simulink model "complete_model"  (R2020b)
settings: Solver=VariableStepAuto  StartTime=0.0  StopTime=10.0  RelTol=1e-3
undefined symbols (not defined in the file or in its folder): D_b_1, D_b_2, D_k_1, D_k_2, D_t_1, D_t_2, E_1, E_2, g, Gs_1, Gs_2, Ix_1, Ix_2, Iy_1, Iy_2, Iz_1, Iz_2, l_1, l_2, m_1, m_2, q_0, q_dot_0
libraries: dspmtrx3 x2, pid_lib x1, dspinverses x1
(part 1 of 2)
settings Model: Creator=lucar  LastModifiedBy=lucar

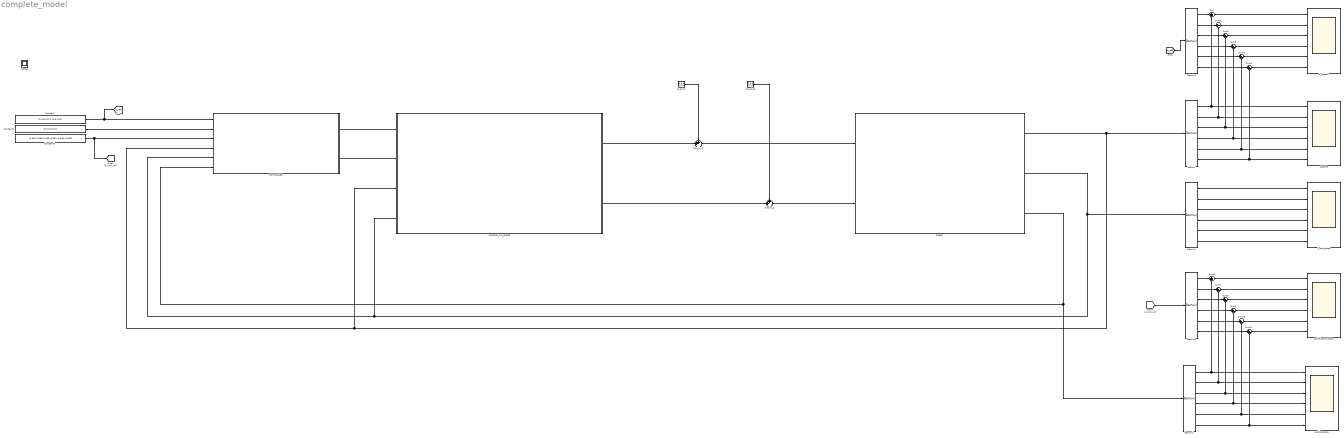
== system complete_model ==
  CONTROLLER : Subsystem
  "CONTROL_TO_FORCE " : Subsystem
  Constant : Constant  Value=[1 0.5 0.3 -1 -0.5 -0.3]
  Constant3 : Constant  Value=[0.001 0.008 0.003 -0.001 -0.005 -0.003]
  Constant4 : Constant  Value=[0 0 0 0 0 0]
  Demux{,1..3,5} (5 alike) : Demux  Outputs=6
  ROBOT : Subsystem
  SUM_W_1 : Sum  Inputs=++|
  SUM_W_2 : Sum  Inputs=++|
  Sum{,1..11} (12 alike) : Sum  Inputs=|+-
  W_ext_1 : Constant  Value=[0 0 0 0 0 0]
  W_ext_21 : Constant  Value=[0 0 0 0 0 0]
  q_ddot_error_scope : Scope  NumInputPorts=6
  q_ddot_scope : Scope  NumInputPorts=6
  q_dot_scope : Scope  NumInputPorts=6
  q_scope : Scope  NumInputPorts=6
  q_scope1 : Scope  NumInputPorts=6
  Scope : Scope
  wires:
  Constant4/1 -> CONTROLLER/2(q_dot_ref)
  "CONTROL_TO_FORCE "/1(W_ctrl_1) -> SUM_W_1/2
  ROBOT/1(q) -> Demux/1, "CONTROL_TO_FORCE "/3(q), CONTROLLER/4(q)
  W_ext_1/1 -> SUM_W_1/1
  W_ext_21/1 -> SUM_W_2/1
  CONTROLLER/1(u_control_1) -> "CONTROL_TO_FORCE "/1(u_ctrl_1)
  CONTROLLER/2(u_control_2) -> "CONTROL_TO_FORCE "/2(u_ctrl_2)
  Constant/1 -> [q_ref], CONTROLLER/1(q_ref)
  SUM_W_2/1 -> ROBOT/2(W2)
  SUM_W_1/1 -> ROBOT/1(W_1)
  "CONTROL_TO_FORCE "/2(W_ctrl_2) -> SUM_W_2/2
  Demux/2 -> q_scope/2, Sum1/2  "b_1"
  Demux/1 -> Sum/2, q_scope/1  "k_1"
  Demux/3 -> q_scope/3, Sum2/2  "t_1"
  Demux/4 -> q_scope/4, Sum3/2  "k_2"
  Demux/5 -> q_scope/5, Sum4/2  "b_2"
  Demux/6 -> q_scope/6, Sum5/2  "t_2"
  Demux1/1 -> q_dot_scope/1  "k_1_dot"
  Demux1/5 -> q_dot_scope/5  "b_2_dot"
  ROBOT/2(q_dot) -> Demux1/1, "CONTROL_TO_FORCE "/4(q_dot), CONTROLLER/5(q_dot)
  Demux1/4 -> q_dot_scope/4  "k_2_dot"
  Demux1/3 -> q_dot_scope/3  "t_1_dot"
  Demux1/2 -> q_dot_scope/2  "b_1_dot"
  Demux1/6 -> q_dot_scope/6  "t_2_dopt"
  Demux3/2 -> Sum1/1  "b_1"
  Demux3/1 -> Sum/1  "k_1"
  Demux3/3 -> Sum2/1  "t_1"
  Demux3/6 -> Sum5/1  "t_2"
  Demux3/4 -> Sum3/1  "k_2"
  Demux3/5 -> Sum4/1  "b_2"
  [q_ref] -> Demux3/1
  Sum5/1 -> q_scope1/6
  Sum4/1 -> q_scope1/5
  Sum3/1 -> q_scope1/4
  Sum2/1 -> q_scope1/3
  Sum1/1 -> q_scope1/2  "b_1_error"
  Sum/1 -> q_scope1/1  "k_1_error"
  ROBOT/3(q_ddot) -> Demux2/1, CONTROLLER/6(q_ddot)
  Demux5/4 -> Sum9/1  "k_2"
  Sum6/1 -> q_ddot_error_scope/1  "k_1_ddot_error"
  Demux5/2 -> Sum7/1  "b_1"
  Demux5/6 -> Sum11/1  "t_2"
  Sum11/1 -> q_ddot_error_scope/6  "t_2_ddot_error"
  Sum9/1 -> q_ddot_error_scope/4  "k_2_ddot_error"
  Demux5/5 -> Sum10/1  "b_2"
  Demux5/3 -> Sum8/1  "t_1"
  Sum8/1 -> q_ddot_error_scope/3  "t_1_ddot_error"
  Sum10/1 -> q_ddot_error_scope/5  "b_2_ddot_error"
  Demux5/1 -> Sum6/1  "k_1"
  Sum7/1 -> q_ddot_error_scope/2  "b_1_ddot_error"
  Demux2/5 -> q_ddot_scope/5, Sum10/2  "b_2_ddot"
  Demux2/3 -> q_ddot_scope/3, Sum8/2  "t_1_ddot"
  Demux2/1 -> q_ddot_scope/1, Sum6/2  "k_1_ddot"
  Demux2/6 -> q_ddot_scope/6, Sum11/2  "t_2_ddot"
  Demux2/2 -> q_ddot_scope/2, Sum7/2  "b_1_ddot"
  Demux2/4 -> q_ddot_scope/4, Sum9/2  "k_2_ddot"
  Constant3/1 -> [q_ddot_ref], CONTROLLER/3(q_ddot_ref)
  [q_ddot_ref] -> Demux5/1

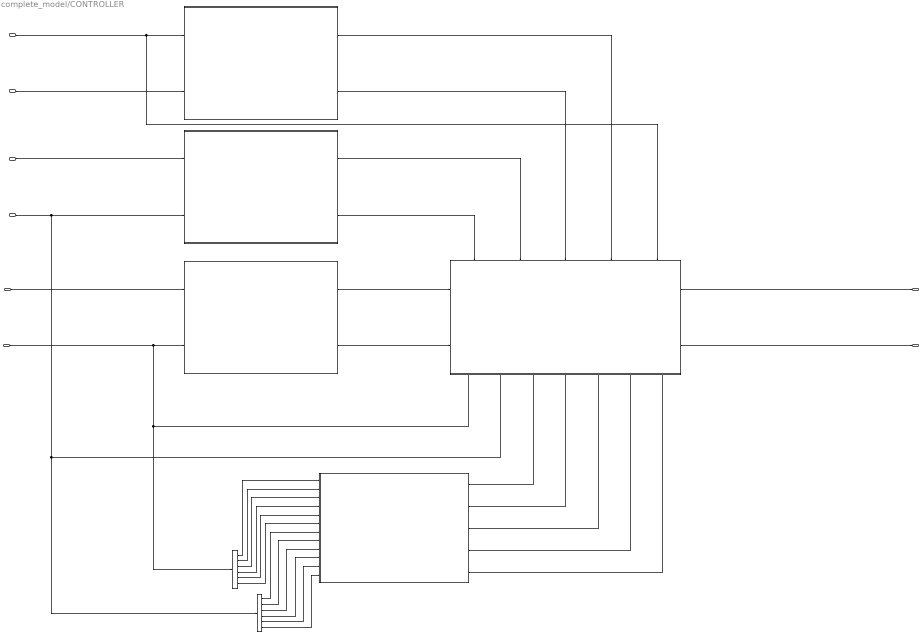
== system complete_model/CONTROLLER ==
  q_ref : Inport
  q_dot_ref : Inport  Port=2
  q_ddot_ref : Inport  Port=3
  q : Inport  Port=4
  q_dot : Inport  Port=5
  q_ddot : Inport  Port=6
  Demux2 : Demux  Outputs=6
  Demux3 : Demux  Outputs=6
  Subsystem : Subsystem
  Subsystem1 : Subsystem
      settings: PortSchema="{\"entries\":[{\"content\":{\"sides\":[{\"content\":{\"connectorIds\":[\"In1\",\"In2\"]},\"type\":\"ConnectorPlacement.EquallySpacedRectSide\",\"uuid\":\"f5a8289a-49c1-4c4e-8602-865d2a4ae65f\"},{\"content\":{\"connectorIds\":[\"Out1\",\"Out2\"],\"side\":\"RIGHT\"},\"type\":\"ConnectorPlacement.EquallySpacedRectSide\",\"uuid\":\"577a7826-c2f6-45a0-b52d-c6289559e493\"},{\"content\":{\"connectorIds\":[\"In3\",\"In4\",\"In5\",\"In6\",\"In7\"],\"side\":\"TOP\"},\"type\":\"ConnectorPlacement.EquallySpacedRectSide\",\"uuid\":\"a36ac755-a99f-4894-9541-2e1b1dc6ecfa\"},{\"content\":{\"connectorIds\":[\"In8\",\"In9\",\"In10\",\"In11\",\"In12\",\"In13\",\"In14\"],\"side\":\"BOTTOM\"},\"type\":\"ConnectorPlacement.EquallySpacedRectSide\",\"uuid\":\"cdbb495b-8222-4370-93c0-90b4d729da35\"},{\"content\":{\"connectorIds\":[],\"side\":\"HIDDEN\"},\"type\":\"ConnectorPlacement.EquallySpacedRectSide\",\"uuid\":\"56f17497-4814-45df-afce-b6f00d804874\"}]},\"type\":\"ConnectorPlacement.EquallySpacedConnector\",\"uuid\":\"c7bc0292-f10c-440d-b55e-954c700d4dfb\"}],\"packageUris\":[\"http://schema.mathworks.com/mf0/Connector/R2020b\"],\"version\":\"1.0\"}"
  Subsystem2 : Subsystem
  Subsystem3 : Subsystem
  Subsystem4 : Subsystem
  u_control_1 : Outport
  u_control_2 : Outport  Port=2
  wires:
  q_ref/1 -> Subsystem/1(In1)
  Subsystem/1(e_1) -> Subsystem1/1(e_1)
  Subsystem/2(e_2) -> Subsystem1/2(e_2)
  Subsystem1/1(u_control_1) -> u_control_1/1
  Subsystem1/2(u_control_2) -> u_control_2/1
  Demux2/6 -> Subsystem2/6(t_2)
  q/1 -> Subsystem/2(In2), Subsystem1/8(q), Demux2/1
  Demux3/3 -> Subsystem2/9(t_dot_1)
  Demux3/1 -> Subsystem2/7(k_dot_1)
  Demux3/2 -> Subsystem2/8(b_dot_1)
  Demux2/4 -> Subsystem2/4(k_2)
  Demux2/2 -> Subsystem2/2(b_1)
  Demux2/1 -> Subsystem2/1(k_1)
  Demux2/3 -> Subsystem2/3(t_1)
  Demux3/5 -> Subsystem2/11(b_dot_2)
  q_dot/1 -> Subsystem1/9(q_dot), Demux3/1, Subsystem3/2(q_dot)
  Demux2/5 -> Subsystem2/5(b_2)
  Demux3/4 -> Subsystem2/10(k_dot_2)
  Demux3/6 -> Subsystem2/12(t_dot_2)
  Subsystem2/1(B) -> Subsystem1/10(B)
  Subsystem2/2(D) -> Subsystem1/11(D)
  Subsystem2/3(C) -> Subsystem1/12(C)
  Subsystem2/4(G) -> Subsystem1/13(G)
  q_dot_ref/1 -> Subsystem3/1(q_dot_ref)
  q_ddot_ref/1 -> Subsystem1/7(q_ddot_ref), Subsystem4/1(q_ddot_ref)
  q_ddot/1 -> Subsystem4/2(q_ddot)
  Subsystem3/2(e_2) -> Subsystem1/3(e_dot_1)
  Subsystem3/1(e_1) -> Subsystem1/4(e_dot_2)
  Subsystem4/2(e_ddot_2) -> Subsystem1/5(e_ddot_1)
  Subsystem4/1(e_ddot_1) -> Subsystem1/6(e_ddot_2)
  Subsystem2/5(G_grav) -> Subsystem1/14(G_grav)

== system complete_model/CONTROL_TO_FORCE  ==
  u_ctrl_1 : Inport
  u_ctrl_2 : Inport  Port=2
  q : Inport  Port=3
  q_dot : Inport  Port=4
  Demux : Demux  Outputs=6
  Demux1 : Demux  Outputs=6
  Subsystem : Subsystem
  W_ctrl_1 : Outport
  W_ctrl_2 : Outport  Port=2
  wires:
  Demux/6 -> Subsystem/8(t_2)
  q/1 -> Demux/1
  Demux1/3 -> Subsystem/11(t_dot_1)
  Demux1/1 -> Subsystem/9(k_dot_1)
  Demux1/2 -> Subsystem/10(b_dot_1)
  Demux/4 -> Subsystem/6(k_2)
  Demux/2 -> Subsystem/4(b_1)
  Demux/1 -> Subsystem/3(k_1)
  Demux/3 -> Subsystem/5(t_1)
  Demux1/5 -> Subsystem/13(b_dot_2)
  q_dot/1 -> Demux1/1
  Demux/5 -> Subsystem/7(b_2)
  Demux1/4 -> Subsystem/12(k_dot_2)
  Demux1/6 -> Subsystem/14(t_dot_2)
  Subsystem/1(W_ctrl_1) -> W_ctrl_1/1
  Subsystem/2(W_ctrl_2) -> W_ctrl_2/1
  u_ctrl_1/1 -> Subsystem/1(u_ctrl_1)
  u_ctrl_2/1 -> Subsystem/2(u_ctrl_2)

== system complete_model/ROBOT ==
  W_1 : Inport
  W2 : Inport  Port=2
  Demux : Demux  Outputs=6
  Demux1 : Demux  Outputs=6
  Integrator : Integrator  InitialCondition=q_dot_0
  Integrator1 : Integrator  InitialCondition=q_0
  Subsystem : Subsystem
  Subsystem1 : Subsystem
  q : Outport
  q_dot : Outport  Port=2
  q_ddot : Outport  Port=3
  wires:
  Subsystem/4(G) -> Subsystem1/5(G)
  Demux/3 -> Subsystem/3(t_1)
  Demux1/6 -> Subsystem/14(t_dot_2)
  Demux1/5 -> Subsystem/13(b_dot_2)
  Demux1/2 -> Subsystem/10(b_dot_1)
  Demux1/4 -> Subsystem/12(k_dot_2)
  Demux/5 -> Subsystem/5(b_2)
  Demux/1 -> Subsystem/1(k_1)
  Subsystem1/1(q_ddot) -> q_ddot/1, Integrator/1
  Demux/4 -> Subsystem/4(k_2)
  Demux1/3 -> Subsystem/11(t_dot_1)
  Demux/2 -> Subsystem/2(b_1)
  Subsystem/1(B) -> Subsystem1/2(B)
  Demux1/1 -> Subsystem/9(k_dot_1)
  Subsystem/3(C) -> Subsystem1/4(C)
  Demux/6 -> Subsystem/6(t_2)
  Subsystem/2(D) -> Subsystem1/3(D)
  W_1/1 -> Subsystem/7(W_1)
  Subsystem/5(U) -> Subsystem1/6(u)
  W2/1 -> Subsystem/8(W_2)
  Integrator1/1 -> q/1, Subsystem1/1(q), Demux/1
  Integrator/1 -> Demux1/1, Subsystem1/7(q_dot), Integrator1/1, q_dot/1

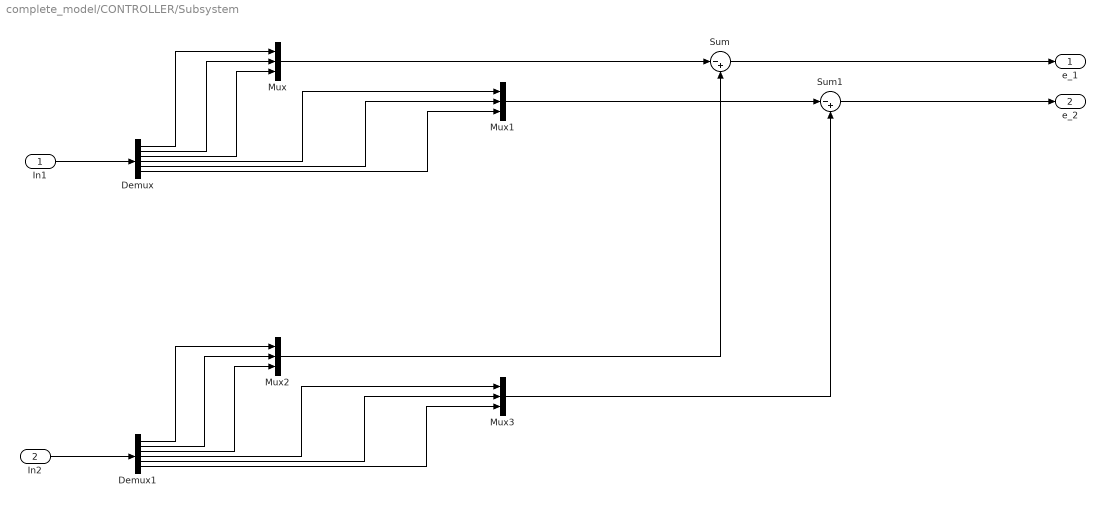
== system complete_model/CONTROLLER/Subsystem ==
  In1 : Inport
  In2 : Inport  Port=2
  Demux : Demux  Outputs=6
  Demux1 : Demux  Outputs=6
  Mux{,1..3} (4 alike) : Mux  Inputs=3
  Sum : Sum  Inputs=|-+
  Sum1 : Sum  Inputs=|-+
  e_1 : Outport
  e_2 : Outport  Port=2
  wires:
  Demux1/6 -> Mux3/3
  Demux/3 -> Mux/3
  Demux1/5 -> Mux3/2
  Demux/2 -> Mux/2
  Mux2/1 -> Sum/2
  Demux/6 -> Mux1/3
  Sum1/1 -> e_2/1
  Demux/1 -> Mux/1
  Demux1/4 -> Mux3/1
  Demux1/3 -> Mux2/3
  Demux1/2 -> Mux2/2
  Demux/5 -> Mux1/2
  Demux1/1 -> Mux2/1
  Sum/1 -> e_1/1
  Mux1/1 -> Sum1/1
  Demux/4 -> Mux1/1
  Mux3/1 -> Sum1/2
  Mux/1 -> Sum/1
  In1/1 -> Demux/1
  In2/1 -> Demux1/1

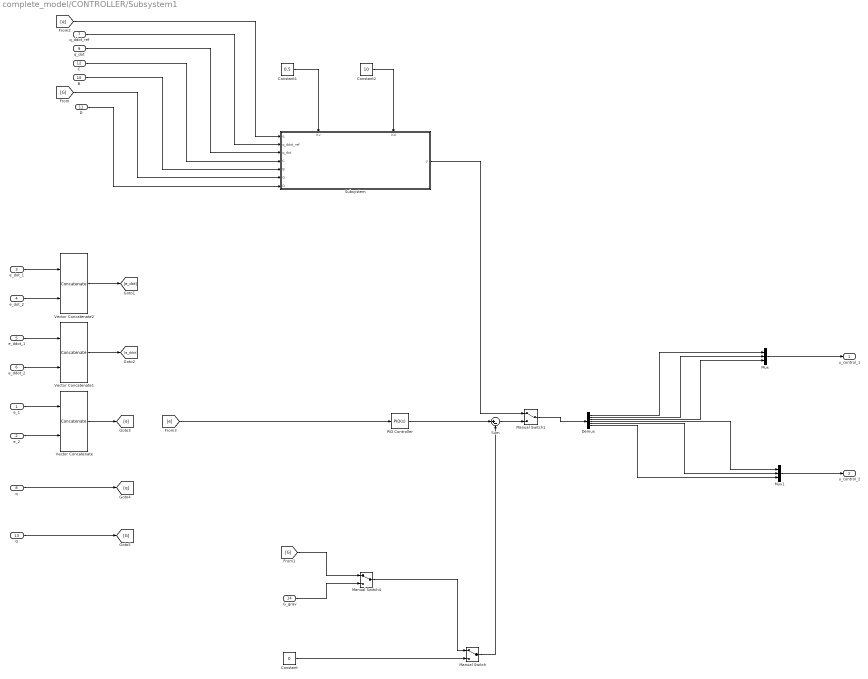
== system complete_model/CONTROLLER/Subsystem1 ==
  e_1 : Inport
  e_2 : Inport  Port=2
  e_dot_1 : Inport  Port=3
  e_dot_2 : Inport  Port=4
  e_ddot_1 : Inport  Port=5
  e_ddot_2 : Inport  Port=6
  q_ddot_ref : Inport  Port=7
  q : Inport  Port=8
  q_dot : Inport  Port=9
  B : Inport  Port=10
  D : Inport  Port=11
  C : Inport  Port=12
  G : Inport  Port=13
  G_grav : Inport  Port=14
  Constant : Constant  Value=0
  Constant1 : Constant  Value=0.5
  Constant2 : Constant  Value=10
  Demux : Demux  Outputs=6
  Manual Switch : ManualSwitch
  Manual Switch1 : ManualSwitch
  Manual Switch4 : ManualSwitch
  Mux : Mux  Inputs=3
  Mux1 : Mux  Inputs=3
  PID Controller : pid_lib/PID Controller  Controller=PID  Form=Parallel  TimeDomain=Continuous-time  UseExternalTs=off  SampleTime=-1  IntegratorMethod=Forward Euler  FilterMethod=Forward Euler  ControllerParametersSource=internal  P=10  I=0  D=0.8  UseFilter=on  N=100  TunerSelectOption=Transfer Function Based (PID Tuner App)  InitialConditionSource=internal  InitialConditionForIntegrator=0  InitialConditionForFilter=0  DifferentiatorICPrevScaledInput=0  ExternalReset=none  TrackingMode=off  Kt=1  LimitOutput=off  SatLimitsSource=internal  UpperSaturationLimit=inf  LowerSaturationLimit=-inf  LinearizeAsGain=on  AntiWindupMode=none  Kb=1  POutMin=[]  POutMax=[]  IOutMin=[]  IOutMax=[]  DOutMin=[]  DOutMax=[]  NOutMin=[]  NOutMax=[]  SumOutMin=[]  SumOutMax=[]  SaturationOutMin=[]  SaturationOutMax=[]  PParamMin=[]  PParamMax=[]  IParamMin=[]  IParamMax=[]  DParamMin=[]  DParamMax=[]  NParamMin=[]  NParamMax=[]  KbParamMin=[]  KbParamMax=[]  KtParamMin=[]  KtParamMax=[]  KbOutMin=[]  KbOutMax=[]  KtOutMin=[]  KtOutMax=[]  IntegratorOutMin=[]  IntegratorOutMax=[]  FilterOutMin=[]  FilterOutMax=[]  SumI1OutMin=[]  SumI1OutMax=[]  SumI2OutMin=[]  SumI2OutMax=[]  SumI3OutMin=[]  SumI3OutMax=[]  SumI4OutMin=[]  SumI4OutMax=[]  SumDOutMin=[]  SumDOutMax=[]  DifferentiatorOutMin=[]  DifferentiatorOutMax=[]  FilterDiffOutCoefMin=[]  FilterDiffOutCoefMax=[]  ReciprocalOutMin=[]  ReciprocalOutMax=[]  SumDenOutMin=[]  SumDenOutMax=[]  SumNumOutMin=[]  SumNumOutMax=[]  DivideOutMin=[]  DivideOutMax=[]  UdiffTsProdOutMin=[]  UdiffTsProdOutMax=[]  NTsProdOutMin=[]  NTsProdOutMax=[]  UintegralTsProdOutMin=[]  UintegralTsProdOutMax=[]  UngainTsProdOutMin=[]  UngainTsProdOutMax=[]  IntegratorContinuousStateAttributes=''  IntegratorStateMustResolveToSignalObject=off  IntegratorRTWStateStorageClass=Auto  FilterContinuousStateAttributes=''  FilterStateMustResolveToSignalObject=off  FilterRTWStateStorageClass=Auto  ParallelPVariant=InternalParameters  IdealPVariant=Disabled  IVariant=InternalParameters  DVariant=InternalParameters  IntegratorVariant=Continuous  SatVariant=Disabled  AWVariant=Passthrough  PCopyVariant=Disabled  TRVariant=Disabled  FdbkBlocksVariant=Forward  IdealPFdbkVariant=Disabled  SatFdbkVariant=Disabled  DerivativeFilterVariant=ContFilter  NVariant=InternalParameters  NCopyVariant=Disabled  FilterICVariant=InternalICsFilter  IntegratorICVariant=InternalICs  ExternalResetVariant=Disabled  TRSumVariant=Passthrough  SumFdbkVariant=Disabled  SumVariant=Sum_PID  TsampFilterVariant=InternalTs  TsampNgainVariant=Passthrough  TsampIntegralVariant=Passthrough  ExternalSaturationOutDataTypeStr=Inherit: Same as second input
  Subsystem : Subsystem
      settings: PortSchema="{\"entries\":[{\"content\":{\"sides\":[{\"content\":{\"connectorIds\":[\"In1\",\"In2\",\"In3\",\"In4\",\"In5\",\"In6\",\"In7\"]},\"type\":\"ConnectorPlacement.EquallySpacedRectSide\",\"uuid\":\"f8378435-2c70-4ca5-b35e-9079000a7188\"},{\"content\":{\"connectorIds\":[\"Out1\"],\"side\":\"RIGHT\"},\"type\":\"ConnectorPlacement.EquallySpacedRectSide\",\"uuid\":\"366e5ae4-a472-4777-8df5-111cdf47ee59\"},{\"content\":{\"connectorIds\":[\"In8\",\"In9\"],\"side\":\"TOP\"},\"type\":\"ConnectorPlacement.EquallySpacedRectSide\",\"uuid\":\"5a70f401-e563-4b1e-a39f-751f70217f1b\"},{\"content\":{\"connectorIds\":[],\"side\":\"HIDDEN\"},\"type\":\"ConnectorPlacement.EquallySpacedRectSide\",\"uuid\":\"6db507d4-eb44-4222-b62b-10b8d3c8cf59\"}]},\"type\":\"ConnectorPlacement.EquallySpacedConnector\",\"uuid\":\"f0240563-1769-4d53-af5c-dad4dbe59b0a\"}],\"packageUris\":[\"http://schema.mathworks.com/mf0/Connector/R2020b\"],\"version\":\"1.0\"}"
  Sum : Sum  Inputs=|+-
  Vector Concatenate : Concatenate
  Vector Concatenate1 : Concatenate
  Vector Concatenate2 : Concatenate
  u_control_1 : Outport
  u_control_2 : Outport  Port=2
  wires:
  e_1/1 -> Vector Concatenate/1
  e_2/1 -> Vector Concatenate/2
  Demux/3 -> Mux/3
  Demux/2 -> Mux/2
  Mux/1 -> u_control_1/1
  Demux/5 -> Mux1/2
  Mux1/1 -> u_control_2/1
  Demux/6 -> Mux1/3
  Demux/1 -> Mux/1
  Demux/4 -> Mux1/1
  Sum/1 -> Manual Switch1/2
  Manual Switch/1 -> Sum/2
  Manual Switch4/1 -> Manual Switch/1
  Constant/1 -> Manual Switch/2
  e_ddot_2/1 -> Vector Concatenate1/2
  e_ddot_1/1 -> Vector Concatenate1/1
  e_dot_2/1 -> Vector Concatenate2/2
  e_dot_1/1 -> Vector Concatenate2/1
  PID Controller/1 -> Sum/1
  Vector Concatenate2/1 -> [e_dot]
  Vector Concatenate1/1 -> [e_ddot]
  Manual Switch1/1 -> Demux/1
  Vector Concatenate/1 -> [e]
  [e] -> PID Controller/1
  q_ddot_ref/1 -> Subsystem/2(q_ddot_ref)
  q_dot/1 -> Subsystem/3(q_dot)
  C/1 -> Subsystem/4(C)
  B/1 -> Subsystem/5(B)
  [G] -> Subsystem/6(G)
  D/1 -> Subsystem/7(D)
  Subsystem/1(y) -> Manual Switch1/1
  Constant1/1 -> Subsystem/8(Kv)
  Constant2/1 -> Subsystem/9(Kd)
  [G] -> Manual Switch4/1
  G_grav/1 -> Manual Switch4/2
  G/1 -> [G]
  q/1 -> [q]
  [q] -> Subsystem/1(q)

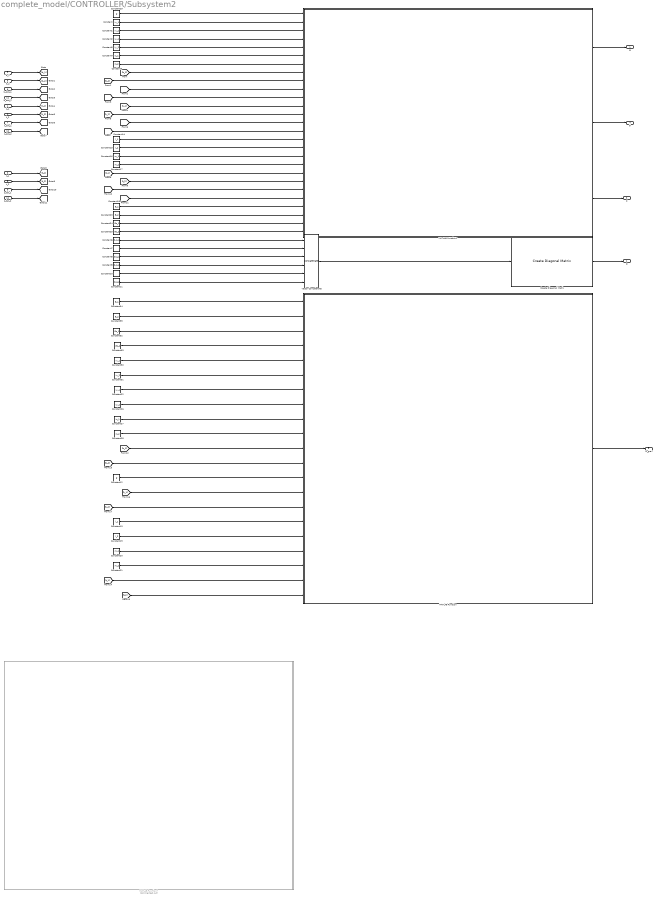
== system complete_model/CONTROLLER/Subsystem2 ==
  k_1 : Inport
  b_1 : Inport  Port=2
  t_1 : Inport  Port=3
  k_2 : Inport  Port=4
  b_2 : Inport  Port=5
  t_2 : Inport  Port=6
  k_dot_1 : Inport  Port=7
  b_dot_1 : Inport  Port=8
  t_dot_1 : Inport  Port=9
  k_dot_2 : Inport  Port=10
  b_dot_2 : Inport  Port=11
  t_dot_2 : Inport  Port=12
  Constant : Constant  Value=Ix_1
  Constant1 : Constant  Value=Ix_2
  Constant10 : Constant  Value=D_b_2
  Constant11 : Constant  Value=D_t_2
  Constant12 : Constant  Value=g
  Constant13 : Constant  Value=l_1
  Constant14 : Constant  Value=l_1
  Constant15 : Constant  Value=l_2
  Constant16 : Constant  Value=m_1
  Constant17 : Constant  Value=m_2
  Constant18 : Constant  Value=E_1
  Constant19 : Constant  Value=l_2
  Constant2 : Constant  Value=Iy_1
  Constant20 : Constant  Value=m_1
  Constant21 : Constant  Value=m_2
  Constant22 : Constant  Value=Iy_1
  Constant23 : Constant  Value=E_2
  Constant24 : Constant  Value=Gs_1
  Constant25 : Constant  Value=Gs_2
  Constant26 : Constant  Value=Iy_2
  Constant27 : Constant  Value=Iz_1
  Constant28 : Constant  Value=Iz_2
  Constant29 : Constant  Value=g
  Constant3 : Constant  Value=Iy_2
  Constant30 : Constant  Value=Ix_1
  Constant31 : Constant  Value=Ix_2
  Constant32 : Constant  Value=Gs_1
  Constant33 : Constant  Value=Gs_2
  Constant34 : Constant  Value=E_1
  Constant35 : Constant  Value=E_2
  Constant4 : Constant  Value=Iz_1
  Constant5 : Constant  Value=Iz_2
  Constant6 : Constant  Value=D_k_1
  Constant7 : Constant  Value=D_b_1
  Constant8 : Constant  Value=D_t_1
  Constant9 : Constant  Value=D_k_2
  Create Diagonal Matrix : dspmtrx3/Create Diagonal Matrix
      settings: SourceProductBaseCode=DS
  MATLAB Function : MATLAB Function  TreatAsAtomicUnit=on
  MATLAB Function1 : Subsystem
      mask help: Simulink:masks:GenSFuncDesc_MD
      mask Help: eval('feval(''rtwprivate'',''rtwhelpview'',''rtw_sfcn_block'')');
  MATLAB Function2 : MATLAB Function  Commented=on  TreatAsAtomicUnit=on
  Vector Concatenate : Concatenate  NumInputs=6
  B : Outport
  D : Outport  Port=2
  C : Outport  Port=3
  G : Outport  Port=4
  G_grav : Outport  Port=5
  wires:
  MATLAB Function1/3(C_matrix) -> C/1
  Constant5/1 -> MATLAB Function1/7(Iz_2)
  Constant18/1 -> MATLAB Function1/24(E_1)
  Constant16/1 -> MATLAB Function1/18(m_1)
  Constant17/1 -> MATLAB Function1/19(m_2)
  Constant25/1 -> MATLAB Function1/27(Gs_2)
  Constant14/1 -> MATLAB Function1/16(l_1)
  Constant1/1 -> MATLAB Function1/3(Ix_2)
  Constant/1 -> MATLAB Function1/2(Ix_1)
  Constant3/1 -> MATLAB Function1/5(Iy_2)
  Constant2/1 -> MATLAB Function1/4(Iy_1)
  Constant4/1 -> MATLAB Function1/6(Iz_1)
  Constant29/1 -> MATLAB Function1/1(g)
  Constant24/1 -> MATLAB Function1/26(Gs_1)
  Constant23/1 -> MATLAB Function1/25(E_2)
  Constant15/1 -> MATLAB Function1/17(l_2)
  MATLAB Function1/1(B_matrix) -> B/1
  MATLAB Function1/2(G_matrix) -> G/1
  Constant7/1 -> Vector Concatenate/2
  Constant6/1 -> Vector Concatenate/1
  Constant8/1 -> Vector Concatenate/3
  Constant9/1 -> Vector Concatenate/4
  Constant10/1 -> Vector Concatenate/5
  Constant11/1 -> Vector Concatenate/6
  Vector Concatenate/1 -> Create Diagonal Matrix/1
  Create Diagonal Matrix/1 -> D/1
  b_1/1 -> [b_1]
  b_2/1 -> [b_2]
  b_dot_1/1 -> [b_dot_1]
  b_dot_2/1 -> [b_dot_2]
  k_1/1 -> [k_1]
  k_2/1 -> [k_2]
  k_dot_1/1 -> [k_dot_1]
  k_dot_2/1 -> [k_dot_2]
  t_2/1 -> [t_2]
  t_dot_2/1 -> [t_dot_2]
  t_1/1 -> [t_1]
  t_dot_1/1 -> [t_dot_1]
  [b_1] -> MATLAB Function1/8(b_1)
  [b_dot_2] -> MATLAB Function1/11(b_dot_2)
  [b_2] -> MATLAB Function1/9(b_2)
  [b_dot_1] -> MATLAB Function1/10(b_dot_1)
  [k_1] -> MATLAB Function1/12(k_1)
  [k_dot_1] -> MATLAB Function1/14(k_dot_1)
  [k_2] -> MATLAB Function1/13(k_2)
  [k_dot_2] -> MATLAB Function1/15(k_dot_2)
  [t_dot_2] -> MATLAB Function1/23(t_dot_2)
  [t_2] -> MATLAB Function1/21(t_2)
  [t_dot_1] -> MATLAB Function1/22(t_dot_1)
  [t_1] -> MATLAB Function1/20(t_1)
  [b_2] -> MATLAB Function/12(b_2)
  [b_1] -> MATLAB Function/11(b_1)
  [t_2] -> MATLAB Function/21(t_2)
  [t_1] -> MATLAB Function/20(t_1)
  Constant12/1 -> MATLAB Function/13(g)
  [k_1] -> MATLAB Function/14(k_1)
  [k_2] -> MATLAB Function/15(k_2)
  Constant19/1 -> MATLAB Function/17(l_2)
  Constant13/1 -> MATLAB Function/16(l_1)
  Constant20/1 -> MATLAB Function/18(m_1)
  Constant21/1 -> MATLAB Function/19(m_2)
  Constant28/1 -> MATLAB Function/10(Iz_2)
  Constant27/1 -> MATLAB Function/9(Iz_1)
  Constant26/1 -> MATLAB Function/8(Iy_2)
  Constant22/1 -> MATLAB Function/7(Iy_1)
  Constant31/1 -> MATLAB Function/6(Ix_2)
  Constant30/1 -> MATLAB Function/5(Ix_1)
  Constant32/1 -> MATLAB Function/3(Gs_1)
  Constant33/1 -> MATLAB Function/4(Gs_2)
  Constant34/1 -> MATLAB Function/1(E_1)
  Constant35/1 -> MATLAB Function/2(E_2)
  MATLAB Function/1(G_g) -> G_grav/1

== system complete_model/CONTROLLER/Subsystem3 ==
  q_dot_ref : Inport
  q_dot : Inport  Port=2
  Demux : Demux  Outputs=6
  Demux1 : Demux  Outputs=6
  Mux{,1..3} (4 alike) : Mux  Inputs=3
  Sum : Sum  Inputs=|-+
  Sum1 : Sum  Inputs=|-+
  e_1 : Outport
  e_2 : Outport  Port=2
  wires:
  Demux1/6 -> Mux3/3
  Demux/3 -> Mux/3
  Demux1/5 -> Mux3/2
  Demux/2 -> Mux/2
  Mux2/1 -> Sum/2
  Demux/6 -> Mux1/3
  Sum1/1 -> e_2/1
  Demux/1 -> Mux/1
  Demux1/4 -> Mux3/1
  Demux1/3 -> Mux2/3
  Demux1/2 -> Mux2/2
  Demux/5 -> Mux1/2
  Demux1/1 -> Mux2/1
  Sum/1 -> e_1/1
  Mux1/1 -> Sum1/1
  Demux/4 -> Mux1/1
  Mux3/1 -> Sum1/2
  Mux/1 -> Sum/1
  q_dot_ref/1 -> Demux/1
  q_dot/1 -> Demux1/1

== system complete_model/CONTROLLER/Subsystem4 ==
  q_ddot_ref : Inport
  q_ddot : Inport  Port=2
  Demux : Demux  Outputs=6
  Demux1 : Demux  Outputs=6
  Mux{,1..3} (4 alike) : Mux  Inputs=3
  Sum : Sum  Inputs=|-+
  Sum1 : Sum  Inputs=|-+
  e_ddot_1 : Outport
  e_ddot_2 : Outport  Port=2
  wires:
  Demux1/6 -> Mux3/3
  Demux/3 -> Mux/3
  Demux1/5 -> Mux3/2
  Demux/2 -> Mux/2
  Mux2/1 -> Sum/2
  Demux/6 -> Mux1/3
  Sum1/1 -> e_ddot_2/1
  Demux/1 -> Mux/1
  Demux1/4 -> Mux3/1
  Demux1/3 -> Mux2/3
  Demux1/2 -> Mux2/2
  Demux/5 -> Mux1/2
  Demux1/1 -> Mux2/1
  Sum/1 -> e_ddot_1/1
  Mux1/1 -> Sum1/1
  Demux/4 -> Mux1/1
  Mux3/1 -> Sum1/2
  Mux/1 -> Sum/1
  q_ddot_ref/1 -> Demux/1
  q_ddot/1 -> Demux1/1

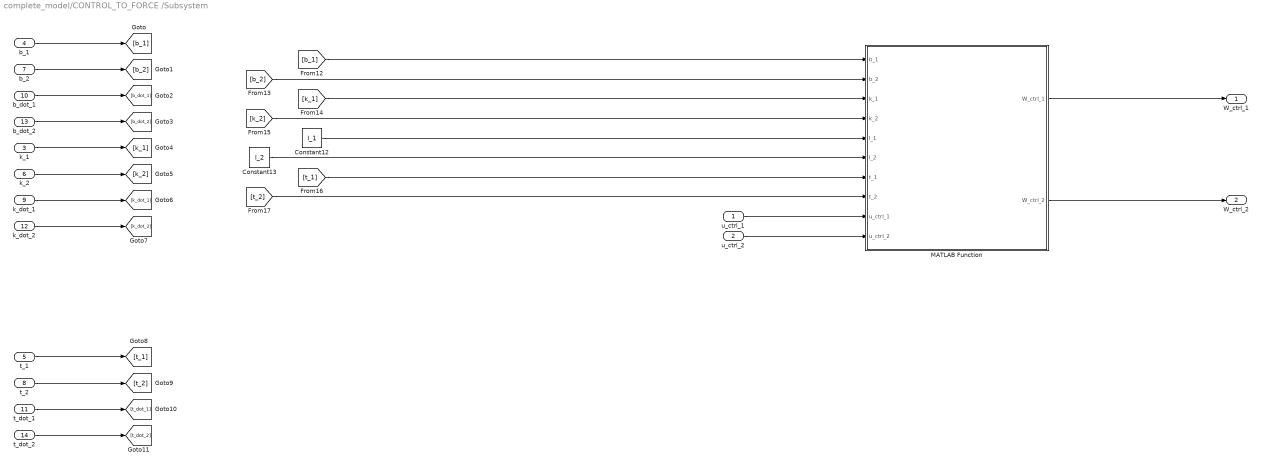
== system complete_model/CONTROL_TO_FORCE /Subsystem ==
  u_ctrl_1 : Inport
  u_ctrl_2 : Inport  Port=2
  k_1 : Inport  Port=3
  b_1 : Inport  Port=4
  t_1 : Inport  Port=5
  k_2 : Inport  Port=6
  b_2 : Inport  Port=7
  t_2 : Inport  Port=8
  k_dot_1 : Inport  Port=9
  b_dot_1 : Inport  Port=10
  t_dot_1 : Inport  Port=11
  k_dot_2 : Inport  Port=12
  b_dot_2 : Inport  Port=13
  t_dot_2 : Inport  Port=14
  Constant12 : Constant  Value=l_1
  Constant13 : Constant  Value=l_2
  MATLAB Function : MATLAB Function  TreatAsAtomicUnit=on
  W_ctrl_1 : Outport  PortDimensions=6
  W_ctrl_2 : Outport  Port=2  PortDimensions=6
  wires:
  u_ctrl_2/1 -> MATLAB Function/10(u_ctrl_2)
  b_2/1 -> [b_2]
  [b_2] -> MATLAB Function/2(b_2)
  t_1/1 -> [t_1]
  [k_2] -> MATLAB Function/4(k_2)
  u_ctrl_1/1 -> MATLAB Function/9(u_ctrl_1)
  t_2/1 -> [t_2]
  k_2/1 -> [k_2]
  t_dot_1/1 -> [t_dot_1]
  Constant13/1 -> MATLAB Function/6(l_2)
  k_dot_1/1 -> [k_dot_1]
  b_1/1 -> [b_1]
  b_dot_2/1 -> [b_dot_2]
  k_dot_2/1 -> [k_dot_2]
  MATLAB Function/1(W_ctrl_1) -> W_ctrl_1/1
  t_dot_2/1 -> [t_dot_2]
  k_1/1 -> [k_1]
  [t_1] -> MATLAB Function/7(t_1)
  b_dot_1/1 -> [b_dot_1]
  [t_2] -> MATLAB Function/8(t_2)
  [k_1] -> MATLAB Function/3(k_1)
  MATLAB Function/2(W_ctrl_2) -> W_ctrl_2/1
  Constant12/1 -> MATLAB Function/5(l_1)
  [b_1] -> MATLAB Function/1(b_1)

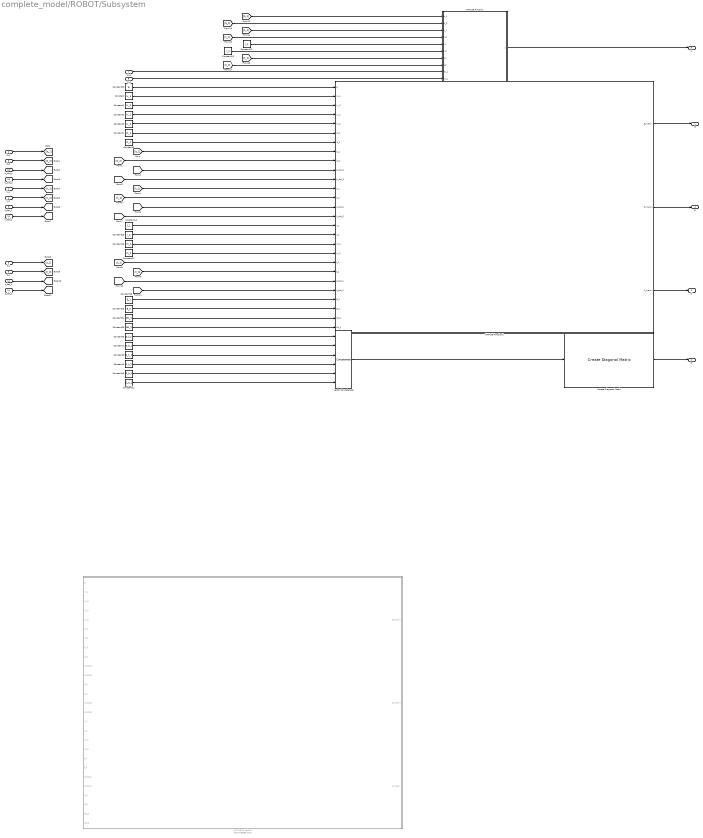
== system complete_model/ROBOT/Subsystem ==
  k_1 : Inport
  b_1 : Inport  Port=2
  t_1 : Inport  Port=3
  k_2 : Inport  Port=4
  b_2 : Inport  Port=5
  t_2 : Inport  Port=6
  W_1 : Inport  Port=7  PortDimensions=6
  W_2 : Inport  Port=8  PortDimensions=6
  k_dot_1 : Inport  Port=9
  b_dot_1 : Inport  Port=10
  t_dot_1 : Inport  Port=11
  k_dot_2 : Inport  Port=12
  b_dot_2 : Inport  Port=13
  t_dot_2 : Inport  Port=14
  Constant : Constant  Value=Ix_1
  Constant1 : Constant  Value=Ix_2
  Constant10 : Constant  Value=D_b_2
  Constant11 : Constant  Value=D_t_2
  Constant12 : Constant  Value=l_1
  Constant13 : Constant  Value=l_2
  Constant14 : Constant  Value=l_1
  Constant15 : Constant  Value=l_2
  Constant16 : Constant  Value=m_1
  Constant17 : Constant  Value=m_2
  Constant18 : Constant  Value=E_1
  Constant2 : Constant  Value=Iy_1
  Constant23 : Constant  Value=E_2
  Constant24 : Constant  Value=Gs_1
  Constant25 : Constant  Value=Gs_2
  Constant29 : Constant  Value=g
  Constant3 : Constant  Value=Iy_2
  Constant4 : Constant  Value=Iz_1
  Constant5 : Constant  Value=Iz_2
  Constant6 : Constant  Value=D_k_1
  Constant7 : Constant  Value=D_b_1
  Constant8 : Constant  Value=D_t_1
  Constant9 : Constant  Value=D_k_2
  Create Diagonal Matrix : dspmtrx3/Create Diagonal Matrix
      settings: SourceProductBaseCode=DS
  MATLAB Function : MATLAB Function  TreatAsAtomicUnit=on
  MATLAB Function1 : Subsystem
      mask help: Simulink:masks:GenSFuncDesc_MD
      mask Help: eval('feval(''rtwprivate'',''rtwhelpview'',''rtw_sfcn_block'')');
  MATLAB Function2 : MATLAB Function  Commented=on  TreatAsAtomicUnit=on
  Vector Concatenate : Concatenate  NumInputs=6
  B : Outport
  D : Outport  Port=2
  C : Outport  Port=3
  G : Outport  Port=4
  U : Outport  Port=5
  wires:
  MATLAB Function1/3(C_matrix) -> C/1
  Constant5/1 -> MATLAB Function1/7(Iz_2)
  Constant18/1 -> MATLAB Function1/24(E_1)
  Constant16/1 -> MATLAB Function1/18(m_1)
  Constant17/1 -> MATLAB Function1/19(m_2)
  Constant25/1 -> MATLAB Function1/27(Gs_2)
  Constant14/1 -> MATLAB Function1/16(l_1)
  Constant1/1 -> MATLAB Function1/3(Ix_2)
  Constant/1 -> MATLAB Function1/2(Ix_1)
  Constant3/1 -> MATLAB Function1/5(Iy_2)
  Constant2/1 -> MATLAB Function1/4(Iy_1)
  Constant4/1 -> MATLAB Function1/6(Iz_1)
  Constant29/1 -> MATLAB Function1/1(g)
  Constant24/1 -> MATLAB Function1/26(Gs_1)
  Constant23/1 -> MATLAB Function1/25(E_2)
  Constant15/1 -> MATLAB Function1/17(l_2)
  MATLAB Function1/1(B_matrix) -> B/1
  MATLAB Function1/2(G_matrix) -> G/1
  Constant7/1 -> Vector Concatenate/2
  Constant6/1 -> Vector Concatenate/1
  Constant8/1 -> Vector Concatenate/3
  Constant9/1 -> Vector Concatenate/4
  Constant10/1 -> Vector Concatenate/5
  Constant11/1 -> Vector Concatenate/6
  Vector Concatenate/1 -> Create Diagonal Matrix/1
  Create Diagonal Matrix/1 -> D/1
  W_1/1 -> MATLAB Function/9(W_1)
  MATLAB Function/1(u) -> U/1
  W_2/1 -> MATLAB Function/10(W_2)
  b_1/1 -> [b_1]
  b_2/1 -> [b_2]
  b_dot_1/1 -> [b_dot_1]
  b_dot_2/1 -> [b_dot_2]
  k_1/1 -> [k_1]
  k_2/1 -> [k_2]
  k_dot_1/1 -> [k_dot_1]
  k_dot_2/1 -> [k_dot_2]
  t_2/1 -> [t_2]
  t_dot_2/1 -> [t_dot_2]
  t_1/1 -> [t_1]
  t_dot_1/1 -> [t_dot_1]
  [b_1] -> MATLAB Function1/8(b_1)
  [b_dot_2] -> MATLAB Function1/11(b_dot_2)
  [b_2] -> MATLAB Function1/9(b_2)
  [b_dot_1] -> MATLAB Function1/10(b_dot_1)
  [k_1] -> MATLAB Function1/12(k_1)
  [k_dot_1] -> MATLAB Function1/14(k_dot_1)
  [k_2] -> MATLAB Function1/13(k_2)
  [k_dot_2] -> MATLAB Function1/15(k_dot_2)
  [t_dot_2] -> MATLAB Function1/23(t_dot_2)
  [t_2] -> MATLAB Function1/21(t_2)
  [t_dot_1] -> MATLAB Function1/22(t_dot_1)
  [t_1] -> MATLAB Function1/20(t_1)
  [b_1] -> MATLAB Function/1(b_1)
  [b_2] -> MATLAB Function/2(b_2)
  [k_1] -> MATLAB Function/3(k_1)
  [k_2] -> MATLAB Function/4(k_2)
  [t_1] -> MATLAB Function/7(t_1)
  [t_2] -> MATLAB Function/8(t_2)
  Constant12/1 -> MATLAB Function/5(l_1)
  Constant13/1 -> MATLAB Function/6(l_2)

== system complete_model/ROBOT/Subsystem1 ==
  q : Inport
  B : Inport  Port=2
  D : Inport  Port=3
  C : Inport  Port=4
  G : Inport  Port=5
  u : Inport  Port=6
  q_dot : Inport  Port=7
  MATLAB Function : MATLAB Function  TreatAsAtomicUnit=on
  Pseudoinverse : dspinverses/Pseudoinverse  wanterr=off  SimulateUsing=Interpreted execution
      settings: SourceProductBaseCode=DS
  q_ddot : Outport
  wires:
  Pseudoinverse/1 -> MATLAB Function/1(inv_B)
  G/1 -> MATLAB Function/4(G)
  C/1 -> MATLAB Function/2(C)
  D/1 -> MATLAB Function/3(D)
  B/1 -> Pseudoinverse/1
  q/1 -> MATLAB Function/6(q)
  MATLAB Function/1(q_ddot) -> q_ddot/1
  q_dot/1 -> MATLAB Function/5(q_dot)
  u/1 -> MATLAB Function/7(u)

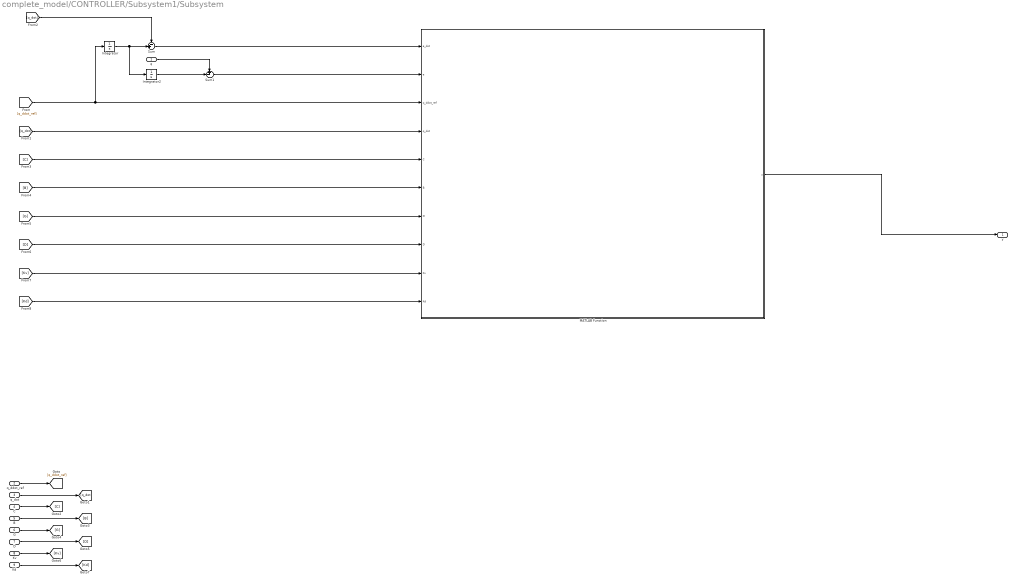
== system complete_model/CONTROLLER/Subsystem1/Subsystem ==
  q : Inport
  q_ddot_ref : Inport  Port=2
  q_dot : Inport  Port=3
  C : Inport  Port=4
  B : Inport  Port=5
  G : Inport  Port=6
  D : Inport  Port=7
  Kv : Inport  Port=8
  Kd : Inport  Port=9
  Integrator : Integrator
  Integrator2 : Integrator
  MATLAB Function : MATLAB Function  TreatAsAtomicUnit=on
  Sum : Sum  Inputs=-+|
  Sum1 : Sum  Inputs=+-|
  y : Outport
  wires:
  MATLAB Function/1(y) -> y/1
  q_ddot_ref/1 -> [q_ddot_ref]
  q_dot/1 -> [q_dot]
  B/1 -> [B]
  D/1 -> [D]
  Kd/1 -> [Kd]
  Kv/1 -> [Kv]
  G/1 -> [G]
  C/1 -> [C]
  [q_ddot_ref] -> Integrator/1, MATLAB Function/3(q_ddot_ref)
  [q_dot] -> MATLAB Function/4(q_dot)
  [q_dot] -> Sum/1
  Integrator/1 -> Integrator2/1, Sum/2
  Sum/1 -> MATLAB Function/1(e_dot)
  Integrator2/1 -> Sum1/2
  [C] -> MATLAB Function/5(C)
  [B] -> MATLAB Function/6(B)
  [G] -> MATLAB Function/7(G)
  [D] -> MATLAB Function/8(D)
  [Kv] -> MATLAB Function/9(Kv)
  [Kd] -> MATLAB Function/10(Kd)
  Sum1/1 -> MATLAB Function/2(e)
  q/1 -> Sum1/1

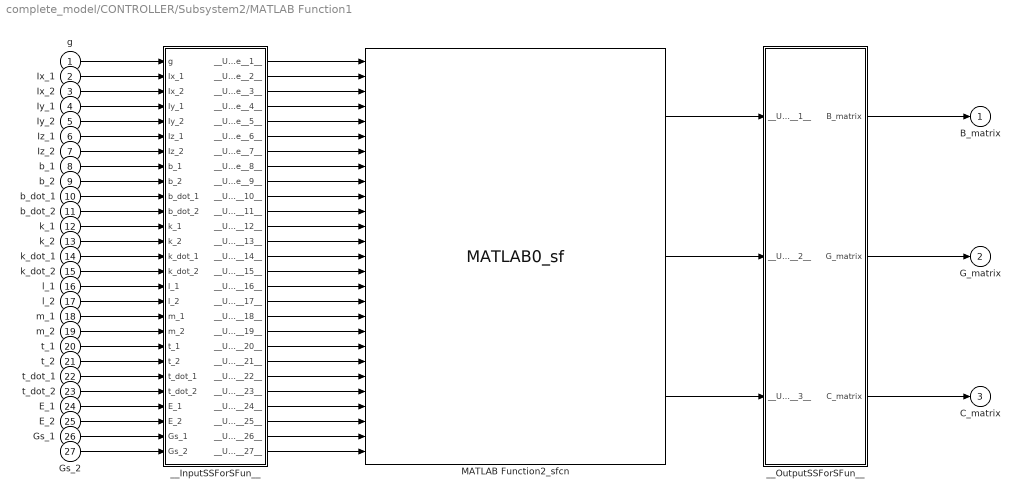
== system complete_model/CONTROLLER/Subsystem2/MATLAB Function1 ==
  g : Inport
  Ix_1 : Inport  Port=2
  Ix_2 : Inport  Port=3
  Iy_1 : Inport  Port=4
  Iy_2 : Inport  Port=5
  Iz_1 : Inport  Port=6
  Iz_2 : Inport  Port=7
  b_1 : Inport  Port=8
  b_2 : Inport  Port=9
  b_dot_1 : Inport  Port=10
  b_dot_2 : Inport  Port=11
  k_1 : Inport  Port=12
  k_2 : Inport  Port=13
  k_dot_1 : Inport  Port=14
  k_dot_2 : Inport  Port=15
  l_1 : Inport  Port=16
  l_2 : Inport  Port=17
  m_1 : Inport  Port=18
  m_2 : Inport  Port=19
  t_1 : Inport  Port=20
  t_2 : Inport  Port=21
  t_dot_1 : Inport  Port=22
  t_dot_2 : Inport  Port=23
  E_1 : Inport  Port=24
  E_2 : Inport  Port=25
  Gs_1 : Inport  Port=26
  Gs_2 : Inport  Port=27
  MATLAB Function2_sfcn : S-Function  FunctionName=MATLAB0_sf  SFunctionModules=""  SFunctionDeploymentMode=off  EnableBusSupport=off  mask{rtw_sf_name=MATLAB0_sf, showVar=off}
      mask prompts: rtw_sf_name "Simulink:masks:GenSFuncName_MP"; showVar "Simulink:masks:GenSFuncShowModuleList_MP"
      mask help: Simulink:masks:GenSFuncDesc_MD
      mask init:
      | displist = '';
      | if ~strcmp(get_param(gcb, 'FunctionName'), rtw_sf_name);
      |   set_param(gcb, 'FunctionName', rtw_sf_name);
      | end
      | % Check if we are generating code
      | rtw_mode = false;
      | if strcmpi(get_param(bdroot(gcb),'SimulationStatus'),'Initializing')
      | 	rtw_mode = strcmpi(get_param(bdroot(gcb),'BuildingRTWCode'),'on') && ...
      | 		~strcmpi(get_param(bdroot(gcb),'TargetStyle'),'SimulationTarget');
      | end
      | if showVar || rtw_mode
      | 	if exist('rtwsfunc') == 2 | exist('rtwsfunc') == 6
      | 		tmplist = rtwsfunc(rtw_sf_name,gcb);
      | 		tmplist = DAStudio.message('Simulink:masks:GenSFuncListOfModules_IC', tmplist);
      | 	elseif showVar
      | 		tmplist1 = DAStudio.message('Simulink:masks:GenSFuncListOfModules_IC', '');
      |         tmplist2 = DAStudio.message('Simulink:masks:GenSFuncNotLicensed_IC');
      |         tmplist = [tmplist1 tmplist2];
      |  	end
      | end
      | if showVar
      |   displist = tmplist;
      | end
      settings: CopyFcn=|
      | if ~strcmp(get_param(gcb,'Linkstatus'),'none') && ...
      | ~strcmp(get_param(gcb,'Linkstatus'),'implicit')
      |   set_param(gcb,'LinkStatus','none');
      | end
      mask Help: eval('feval(''rtwprivate'',''rtwhelpview'',''rtw_sfcn_block'')');
      mask Display:
      | port_label('input',1,'g');
      | port_label('input',2,'Ix_1');
      | port_label('input',3,'Ix_2');
      | port_label('input',4,'Iy_1');
      | port_label('input',5,'Iy_2');
      | port_label('input',6,'Iz_1');
      | port_label('input',7,'Iz_2');
      | port_label('input',8,'b_1');
      | port_label('input',9,'b_2');
      | port_label('input',10,'b_dot_1');
      | port_label('input',11,'b_dot_2');
      | port_label('input',12,'k_1');
      | port_label('input',13,'k_2');
      | port_label('input',14,'k_dot_1');
      | port_label('input',15,'k_dot_2');
      | port_label('input',16,'l_1');
      | port_label('input',17,'l_2');
      | port_label('input',18,'m_1');
      | port_label('input',19,'m_2');
      | port_label('input',20,'t_1');
      | port_label('input',21,'t_2');
      | port_label('input',22,'t_dot_1');
      | port_label('input',23,'t_dot_2');
      | port_label('input',24,'E_1');
      | port_label('input',25,'E_2');
      | port_label('input',26,'Gs_1');
      | port_label('input',27,'Gs_2');
      | port_label('output',1,'B_matrix');
      | port_label('output',2,'G_matrix');
      | port_label('output',3,'C_matrix');
  __InputSSForSFun__ : Subsystem
  __OutputSSForSFun__ : Subsystem
  B_matrix : Outport
  G_matrix : Outport  Port=2
  C_matrix : Outport  Port=3
  wires:
  g/1 -> __InputSSForSFun__/1(g)
  Ix_1/1 -> __InputSSForSFun__/2(Ix_1)
  Ix_2/1 -> __InputSSForSFun__/3(Ix_2)
  Iy_1/1 -> __InputSSForSFun__/4(Iy_1)
  Iy_2/1 -> __InputSSForSFun__/5(Iy_2)
  Iz_1/1 -> __InputSSForSFun__/6(Iz_1)
  Iz_2/1 -> __InputSSForSFun__/7(Iz_2)
  b_1/1 -> __InputSSForSFun__/8(b_1)
  b_2/1 -> __InputSSForSFun__/9(b_2)
  b_dot_1/1 -> __InputSSForSFun__/10(b_dot_1)
  b_dot_2/1 -> __InputSSForSFun__/11(b_dot_2)
  k_1/1 -> __InputSSForSFun__/12(k_1)
  k_2/1 -> __InputSSForSFun__/13(k_2)
  k_dot_1/1 -> __InputSSForSFun__/14(k_dot_1)
  k_dot_2/1 -> __InputSSForSFun__/15(k_dot_2)
  l_1/1 -> __InputSSForSFun__/16(l_1)
  l_2/1 -> __InputSSForSFun__/17(l_2)
  m_1/1 -> __InputSSForSFun__/18(m_1)
  m_2/1 -> __InputSSForSFun__/19(m_2)
  t_1/1 -> __InputSSForSFun__/20(t_1)
  t_2/1 -> __InputSSForSFun__/21(t_2)
  t_dot_1/1 -> __InputSSForSFun__/22(t_dot_1)
  t_dot_2/1 -> __InputSSForSFun__/23(t_dot_2)
  E_1/1 -> __InputSSForSFun__/24(E_1)
  E_2/1 -> __InputSSForSFun__/25(E_2)
  Gs_1/1 -> __InputSSForSFun__/26(Gs_1)
  Gs_2/1 -> __InputSSForSFun__/27(Gs_2)
  __InputSSForSFun__/1(__UniqueOutportName__1__) -> MATLAB Function2_sfcn/1
  __InputSSForSFun__/2(__UniqueOutportName__2__) -> MATLAB Function2_sfcn/2
  __InputSSForSFun__/3(__UniqueOutportName__3__) -> MATLAB Function2_sfcn/3
  __InputSSForSFun__/4(__UniqueOutportName__4__) -> MATLAB Function2_sfcn/4
  __InputSSForSFun__/5(__UniqueOutportName__5__) -> MATLAB Function2_sfcn/5
  __InputSSForSFun__/6(__UniqueOutportName__6__) -> MATLAB Function2_sfcn/6
  __InputSSForSFun__/7(__UniqueOutportName__7__) -> MATLAB Function2_sfcn/7
  __InputSSForSFun__/8(__UniqueOutportName__8__) -> MATLAB Function2_sfcn/8
  __InputSSForSFun__/9(__UniqueOutportName__9__) -> MATLAB Function2_sfcn/9
  __InputSSForSFun__/10(__UniqueOutportName__10__) -> MATLAB Function2_sfcn/10
  __InputSSForSFun__/11(__UniqueOutportName__11__) -> MATLAB Function2_sfcn/11
  __InputSSForSFun__/12(__UniqueOutportName__12__) -> MATLAB Function2_sfcn/12
  __InputSSForSFun__/13(__UniqueOutportName__13__) -> MATLAB Function2_sfcn/13
  __InputSSForSFun__/14(__UniqueOutportName__14__) -> MATLAB Function2_sfcn/14
  __InputSSForSFun__/15(__UniqueOutportName__15__) -> MATLAB Function2_sfcn/15
  __InputSSForSFun__/16(__UniqueOutportName__16__) -> MATLAB Function2_sfcn/16
  __InputSSForSFun__/17(__UniqueOutportName__17__) -> MATLAB Function2_sfcn/17
  __InputSSForSFun__/18(__UniqueOutportName__18__) -> MATLAB Function2_sfcn/18
  __InputSSForSFun__/19(__UniqueOutportName__19__) -> MATLAB Function2_sfcn/19
  __InputSSForSFun__/20(__UniqueOutportName__20__) -> MATLAB Function2_sfcn/20
  __InputSSForSFun__/21(__UniqueOutportName__21__) -> MATLAB Function2_sfcn/21
  __InputSSForSFun__/22(__UniqueOutportName__22__) -> MATLAB Function2_sfcn/22
  __InputSSForSFun__/23(__UniqueOutportName__23__) -> MATLAB Function2_sfcn/23
  __InputSSForSFun__/24(__UniqueOutportName__24__) -> MATLAB Function2_sfcn/24
  __InputSSForSFun__/25(__UniqueOutportName__25__) -> MATLAB Function2_sfcn/25
  __InputSSForSFun__/26(__UniqueOutportName__26__) -> MATLAB Function2_sfcn/26
  __InputSSForSFun__/27(__UniqueOutportName__27__) -> MATLAB Function2_sfcn/27
  MATLAB Function2_sfcn/1 -> __OutputSSForSFun__/1(__UniqueInportName__1__)
  MATLAB Function2_sfcn/2 -> __OutputSSForSFun__/2(__UniqueInportName__2__)
  MATLAB Function2_sfcn/3 -> __OutputSSForSFun__/3(__UniqueInportName__3__)
  __OutputSSForSFun__/1(B_matrix) -> B_matrix/1
  __OutputSSForSFun__/2(G_matrix) -> G_matrix/1
  __OutputSSForSFun__/3(C_matrix) -> C_matrix/1

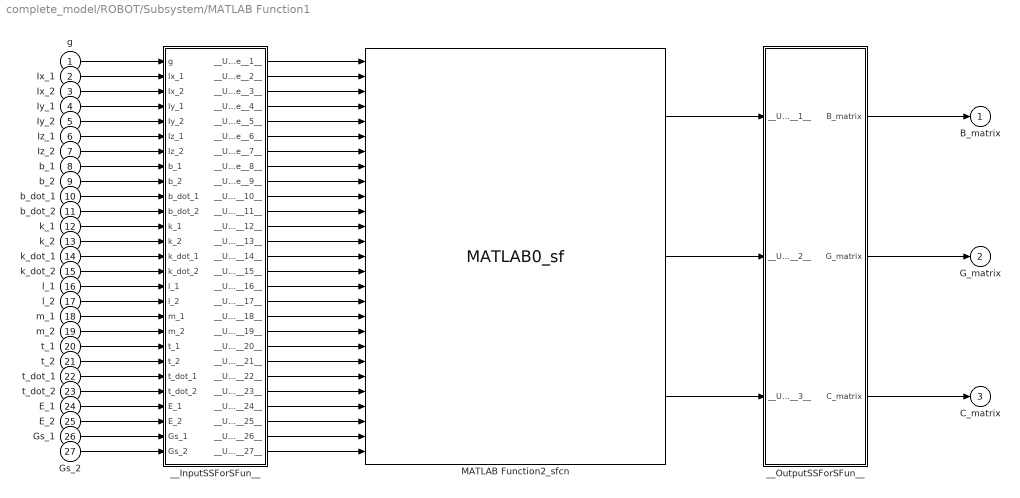
== system complete_model/ROBOT/Subsystem/MATLAB Function1 ==
  g : Inport
  Ix_1 : Inport  Port=2
  Ix_2 : Inport  Port=3
  Iy_1 : Inport  Port=4
  Iy_2 : Inport  Port=5
  Iz_1 : Inport  Port=6
  Iz_2 : Inport  Port=7
  b_1 : Inport  Port=8
  b_2 : Inport  Port=9
  b_dot_1 : Inport  Port=10
  b_dot_2 : Inport  Port=11
  k_1 : Inport  Port=12
  k_2 : Inport  Port=13
  k_dot_1 : Inport  Port=14
  k_dot_2 : Inport  Port=15
  l_1 : Inport  Port=16
  l_2 : Inport  Port=17
  m_1 : Inport  Port=18
  m_2 : Inport  Port=19
  t_1 : Inport  Port=20
  t_2 : Inport  Port=21
  t_dot_1 : Inport  Port=22
  t_dot_2 : Inport  Port=23
  E_1 : Inport  Port=24
  E_2 : Inport  Port=25
  Gs_1 : Inport  Port=26
  Gs_2 : Inport  Port=27
  MATLAB Function2_sfcn : S-Function  FunctionName=MATLAB0_sf  SFunctionModules=""  SFunctionDeploymentMode=off  EnableBusSupport=off  mask{rtw_sf_name=MATLAB0_sf, showVar=off}
      mask prompts: rtw_sf_name "Simulink:masks:GenSFuncName_MP"; showVar "Simulink:masks:GenSFuncShowModuleList_MP"
      mask help: Simulink:masks:GenSFuncDesc_MD
      mask init: same as complete_model/CONTROLLER/Subsystem2/MATLAB Function1/MATLAB Function2_sfcn
      settings: CopyFcn=|
      | if ~strcmp(get_param(gcb,'Linkstatus'),'none') && ...
      | ~strcmp(get_param(gcb,'Linkstatus'),'implicit')
      |   set_param(gcb,'LinkStatus','none');
      | end
      mask Help: eval('feval(''rtwprivate'',''rtwhelpview'',''rtw_sfcn_block'')');
      mask Display:
      | port_label('input',1,'g');
      | port_label('input',2,'Ix_1');
      | port_label('input',3,'Ix_2');
      | port_label('input',4,'Iy_1');
      | port_label('input',5,'Iy_2');
      | port_label('input',6,'Iz_1');
      | port_label('input',7,'Iz_2');
      | port_label('input',8,'b_1');
      | port_label('input',9,'b_2');
      | port_label('input',10,'b_dot_1');
      | port_label('input',11,'b_dot_2');
      | port_label('input',12,'k_1');
      | port_label('input',13,'k_2');
      | port_label('input',14,'k_dot_1');
      | port_label('input',15,'k_dot_2');
      | port_label('input',16,'l_1');
      | port_label('input',17,'l_2');
      | port_label('input',18,'m_1');
      | port_label('input',19,'m_2');
      | port_label('input',20,'t_1');
      | port_label('input',21,'t_2');
      | port_label('input',22,'t_dot_1');
      | port_label('input',23,'t_dot_2');
      | port_label('input',24,'E_1');
      | port_label('input',25,'E_2');
      | port_label('input',26,'Gs_1');
      | port_label('input',27,'Gs_2');
      | port_label('output',1,'B_matrix');
      | port_label('output',2,'G_matrix');
      | port_label('output',3,'C_matrix');
  __InputSSForSFun__ : Subsystem
  __OutputSSForSFun__ : Subsystem
  B_matrix : Outport
  G_matrix : Outport  Port=2
  C_matrix : Outport  Port=3
  wires:
  g/1 -> __InputSSForSFun__/1(g)
  Ix_1/1 -> __InputSSForSFun__/2(Ix_1)
  Ix_2/1 -> __InputSSForSFun__/3(Ix_2)
  Iy_1/1 -> __InputSSForSFun__/4(Iy_1)
  Iy_2/1 -> __InputSSForSFun__/5(Iy_2)
  Iz_1/1 -> __InputSSForSFun__/6(Iz_1)
  Iz_2/1 -> __InputSSForSFun__/7(Iz_2)
  b_1/1 -> __InputSSForSFun__/8(b_1)
  b_2/1 -> __InputSSForSFun__/9(b_2)
  b_dot_1/1 -> __InputSSForSFun__/10(b_dot_1)
  b_dot_2/1 -> __InputSSForSFun__/11(b_dot_2)
  k_1/1 -> __InputSSForSFun__/12(k_1)
  k_2/1 -> __InputSSForSFun__/13(k_2)
  k_dot_1/1 -> __InputSSForSFun__/14(k_dot_1)
  k_dot_2/1 -> __InputSSForSFun__/15(k_dot_2)
  l_1/1 -> __InputSSForSFun__/16(l_1)
  l_2/1 -> __InputSSForSFun__/17(l_2)
  m_1/1 -> __InputSSForSFun__/18(m_1)
  m_2/1 -> __InputSSForSFun__/19(m_2)
  t_1/1 -> __InputSSForSFun__/20(t_1)
  t_2/1 -> __InputSSForSFun__/21(t_2)
  t_dot_1/1 -> __InputSSForSFun__/22(t_dot_1)
  t_dot_2/1 -> __InputSSForSFun__/23(t_dot_2)
  E_1/1 -> __InputSSForSFun__/24(E_1)
  E_2/1 -> __InputSSForSFun__/25(E_2)
  Gs_1/1 -> __InputSSForSFun__/26(Gs_1)
  Gs_2/1 -> __InputSSForSFun__/27(Gs_2)
  __InputSSForSFun__/1(__UniqueOutportName__1__) -> MATLAB Function2_sfcn/1
  __InputSSForSFun__/2(__UniqueOutportName__2__) -> MATLAB Function2_sfcn/2
  __InputSSForSFun__/3(__UniqueOutportName__3__) -> MATLAB Function2_sfcn/3
  __InputSSForSFun__/4(__UniqueOutportName__4__) -> MATLAB Function2_sfcn/4
  __InputSSForSFun__/5(__UniqueOutportName__5__) -> MATLAB Function2_sfcn/5
  __InputSSForSFun__/6(__UniqueOutportName__6__) -> MATLAB Function2_sfcn/6
  __InputSSForSFun__/7(__UniqueOutportName__7__) -> MATLAB Function2_sfcn/7
  __InputSSForSFun__/8(__UniqueOutportName__8__) -> MATLAB Function2_sfcn/8
  __InputSSForSFun__/9(__UniqueOutportName__9__) -> MATLAB Function2_sfcn/9
  __InputSSForSFun__/10(__UniqueOutportName__10__) -> MATLAB Function2_sfcn/10
  __InputSSForSFun__/11(__UniqueOutportName__11__) -> MATLAB Function2_sfcn/11
  __InputSSForSFun__/12(__UniqueOutportName__12__) -> MATLAB Function2_sfcn/12
  __InputSSForSFun__/13(__UniqueOutportName__13__) -> MATLAB Function2_sfcn/13
  __InputSSForSFun__/14(__UniqueOutportName__14__) -> MATLAB Function2_sfcn/14
  __InputSSForSFun__/15(__UniqueOutportName__15__) -> MATLAB Function2_sfcn/15
  __InputSSForSFun__/16(__UniqueOutportName__16__) -> MATLAB Function2_sfcn/16
  __InputSSForSFun__/17(__UniqueOutportName__17__) -> MATLAB Function2_sfcn/17
  __InputSSForSFun__/18(__UniqueOutportName__18__) -> MATLAB Function2_sfcn/18
  __InputSSForSFun__/19(__UniqueOutportName__19__) -> MATLAB Function2_sfcn/19
  __InputSSForSFun__/20(__UniqueOutportName__20__) -> MATLAB Function2_sfcn/20
  __InputSSForSFun__/21(__UniqueOutportName__21__) -> MATLAB Function2_sfcn/21
  __InputSSForSFun__/22(__UniqueOutportName__22__) -> MATLAB Function2_sfcn/22
  __InputSSForSFun__/23(__UniqueOutportName__23__) -> MATLAB Function2_sfcn/23
  __InputSSForSFun__/24(__UniqueOutportName__24__) -> MATLAB Function2_sfcn/24
  __InputSSForSFun__/25(__UniqueOutportName__25__) -> MATLAB Function2_sfcn/25
  __InputSSForSFun__/26(__UniqueOutportName__26__) -> MATLAB Function2_sfcn/26
  __InputSSForSFun__/27(__UniqueOutportName__27__) -> MATLAB Function2_sfcn/27
  MATLAB Function2_sfcn/1 -> __OutputSSForSFun__/1(__UniqueInportName__1__)
  MATLAB Function2_sfcn/2 -> __OutputSSForSFun__/2(__UniqueInportName__2__)
  MATLAB Function2_sfcn/3 -> __OutputSSForSFun__/3(__UniqueInportName__3__)
  __OutputSSForSFun__/1(B_matrix) -> B_matrix/1
  __OutputSSForSFun__/2(G_matrix) -> G_matrix/1
  __OutputSSForSFun__/3(C_matrix) -> C_matrix/1

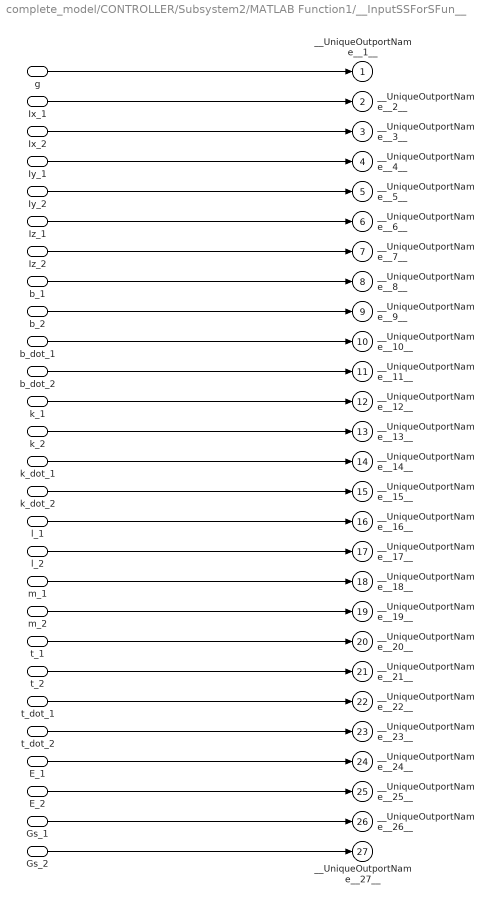
== system complete_model/CONTROLLER/Subsystem2/MATLAB Function1/__InputSSForSFun__ ==
  g : Inport
  Ix_1 : Inport  Port=2
  Ix_2 : Inport  Port=3
  Iy_1 : Inport  Port=4
  Iy_2 : Inport  Port=5
  Iz_1 : Inport  Port=6
  Iz_2 : Inport  Port=7
  b_1 : Inport  Port=8
  b_2 : Inport  Port=9
  b_dot_1 : Inport  Port=10
  b_dot_2 : Inport  Port=11
  k_1 : Inport  Port=12
  k_2 : Inport  Port=13
  k_dot_1 : Inport  Port=14
  k_dot_2 : Inport  Port=15
  l_1 : Inport  Port=16
  l_2 : Inport  Port=17
  m_1 : Inport  Port=18
  m_2 : Inport  Port=19
  t_1 : Inport  Port=20
  t_2 : Inport  Port=21
  t_dot_1 : Inport  Port=22
  t_dot_2 : Inport  Port=23
  E_1 : Inport  Port=24
  E_2 : Inport  Port=25
  Gs_1 : Inport  Port=26
  Gs_2 : Inport  Port=27
  __UniqueOutportName__1__ : Outport
  __UniqueOutportName__2__ : Outport  Port=2
  __UniqueOutportName__3__ : Outport  Port=3
  __UniqueOutportName__4__ : Outport  Port=4
  __UniqueOutportName__5__ : Outport  Port=5
  __UniqueOutportName__6__ : Outport  Port=6
  __UniqueOutportName__7__ : Outport  Port=7
  __UniqueOutportName__8__ : Outport  Port=8
  __UniqueOutportName__9__ : Outport  Port=9
  __UniqueOutportName__10__ : Outport  Port=10
  __UniqueOutportName__11__ : Outport  Port=11
  __UniqueOutportName__12__ : Outport  Port=12
  __UniqueOutportName__13__ : Outport  Port=13
  __UniqueOutportName__14__ : Outport  Port=14
  __UniqueOutportName__15__ : Outport  Port=15
  __UniqueOutportName__16__ : Outport  Port=16
  __UniqueOutportName__17__ : Outport  Port=17
  __UniqueOutportName__18__ : Outport  Port=18
  __UniqueOutportName__19__ : Outport  Port=19
  __UniqueOutportName__20__ : Outport  Port=20
  __UniqueOutportName__21__ : Outport  Port=21
  __UniqueOutportName__22__ : Outport  Port=22
  __UniqueOutportName__23__ : Outport  Port=23
  __UniqueOutportName__24__ : Outport  Port=24
  __UniqueOutportName__25__ : Outport  Port=25
  __UniqueOutportName__26__ : Outport  Port=26
  __UniqueOutportName__27__ : Outport  Port=27
  wires:
  g/1 -> __UniqueOutportName__1__/1
  Ix_1/1 -> __UniqueOutportName__2__/1
  Ix_2/1 -> __UniqueOutportName__3__/1
  Iy_1/1 -> __UniqueOutportName__4__/1
  Iy_2/1 -> __UniqueOutportName__5__/1
  Iz_1/1 -> __UniqueOutportName__6__/1
  Iz_2/1 -> __UniqueOutportName__7__/1
  b_1/1 -> __UniqueOutportName__8__/1
  b_2/1 -> __UniqueOutportName__9__/1
  b_dot_1/1 -> __UniqueOutportName__10__/1
  b_dot_2/1 -> __UniqueOutportName__11__/1
  k_1/1 -> __UniqueOutportName__12__/1
  k_2/1 -> __UniqueOutportName__13__/1
  k_dot_1/1 -> __UniqueOutportName__14__/1
  k_dot_2/1 -> __UniqueOutportName__15__/1
  l_1/1 -> __UniqueOutportName__16__/1
  l_2/1 -> __UniqueOutportName__17__/1
  m_1/1 -> __UniqueOutportName__18__/1
  m_2/1 -> __UniqueOutportName__19__/1
  t_1/1 -> __UniqueOutportName__20__/1
  t_2/1 -> __UniqueOutportName__21__/1
  t_dot_1/1 -> __UniqueOutportName__22__/1
  t_dot_2/1 -> __UniqueOutportName__23__/1
  E_1/1 -> __UniqueOutportName__24__/1
  E_2/1 -> __UniqueOutportName__25__/1
  Gs_1/1 -> __UniqueOutportName__26__/1
  Gs_2/1 -> __UniqueOutportName__27__/1

== system complete_model/CONTROLLER/Subsystem2/MATLAB Function1/__OutputSSForSFun__ ==
  __UniqueInportName__1__ : Inport
  __UniqueInportName__2__ : Inport  Port=2
  __UniqueInportName__3__ : Inport  Port=3
  B_matrix : Outport
  G_matrix : Outport  Port=2
  C_matrix : Outport  Port=3
  wires:
  __UniqueInportName__1__/1 -> B_matrix/1  "B_matrix"
  __UniqueInportName__2__/1 -> G_matrix/1  "G_matrix"
  __UniqueInportName__3__/1 -> C_matrix/1  "C_matrix"

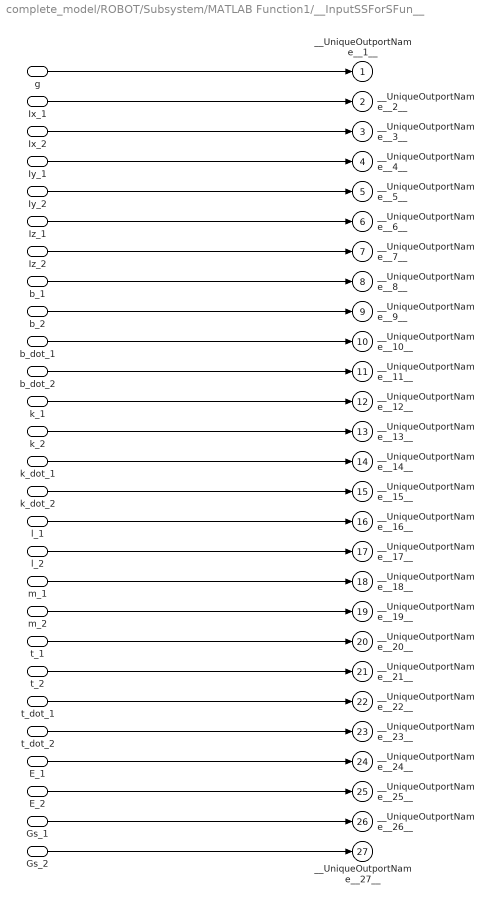
== system complete_model/ROBOT/Subsystem/MATLAB Function1/__InputSSForSFun__ ==
  g : Inport
  Ix_1 : Inport  Port=2
  Ix_2 : Inport  Port=3
  Iy_1 : Inport  Port=4
  Iy_2 : Inport  Port=5
  Iz_1 : Inport  Port=6
  Iz_2 : Inport  Port=7
  b_1 : Inport  Port=8
  b_2 : Inport  Port=9
  b_dot_1 : Inport  Port=10
  b_dot_2 : Inport  Port=11
  k_1 : Inport  Port=12
  k_2 : Inport  Port=13
  k_dot_1 : Inport  Port=14
  k_dot_2 : Inport  Port=15
  l_1 : Inport  Port=16
  l_2 : Inport  Port=17
  m_1 : Inport  Port=18
  m_2 : Inport  Port=19
  t_1 : Inport  Port=20
  t_2 : Inport  Port=21
  t_dot_1 : Inport  Port=22
  t_dot_2 : Inport  Port=23
  E_1 : Inport  Port=24
  E_2 : Inport  Port=25
  Gs_1 : Inport  Port=26
  Gs_2 : Inport  Port=27
  __UniqueOutportName__1__ : Outport
  __UniqueOutportName__2__ : Outport  Port=2
  __UniqueOutportName__3__ : Outport  Port=3
  __UniqueOutportName__4__ : Outport  Port=4
  __UniqueOutportName__5__ : Outport  Port=5
  __UniqueOutportName__6__ : Outport  Port=6
  __UniqueOutportName__7__ : Outport  Port=7
  __UniqueOutportName__8__ : Outport  Port=8
  __UniqueOutportName__9__ : Outport  Port=9
  __UniqueOutportName__10__ : Outport  Port=10
  __UniqueOutportName__11__ : Outport  Port=11
  __UniqueOutportName__12__ : Outport  Port=12
  __UniqueOutportName__13__ : Outport  Port=13
  __UniqueOutportName__14__ : Outport  Port=14
  __UniqueOutportName__15__ : Outport  Port=15
  __UniqueOutportName__16__ : Outport  Port=16
  __UniqueOutportName__17__ : Outport  Port=17
  __UniqueOutportName__18__ : Outport  Port=18
  __UniqueOutportName__19__ : Outport  Port=19
  __UniqueOutportName__20__ : Outport  Port=20
  __UniqueOutportName__21__ : Outport  Port=21
  __UniqueOutportName__22__ : Outport  Port=22
  __UniqueOutportName__23__ : Outport  Port=23
  __UniqueOutportName__24__ : Outport  Port=24
  __UniqueOutportName__25__ : Outport  Port=25
  __UniqueOutportName__26__ : Outport  Port=26
  __UniqueOutportName__27__ : Outport  Port=27
  wires:
  g/1 -> __UniqueOutportName__1__/1
  Ix_1/1 -> __UniqueOutportName__2__/1
  Ix_2/1 -> __UniqueOutportName__3__/1
  Iy_1/1 -> __UniqueOutportName__4__/1
  Iy_2/1 -> __UniqueOutportName__5__/1
  Iz_1/1 -> __UniqueOutportName__6__/1
  Iz_2/1 -> __UniqueOutportName__7__/1
  b_1/1 -> __UniqueOutportName__8__/1
  b_2/1 -> __UniqueOutportName__9__/1
  b_dot_1/1 -> __UniqueOutportName__10__/1
  b_dot_2/1 -> __UniqueOutportName__11__/1
  k_1/1 -> __UniqueOutportName__12__/1
  k_2/1 -> __UniqueOutportName__13__/1
  k_dot_1/1 -> __UniqueOutportName__14__/1
  k_dot_2/1 -> __UniqueOutportName__15__/1
  l_1/1 -> __UniqueOutportName__16__/1
  l_2/1 -> __UniqueOutportName__17__/1
  m_1/1 -> __UniqueOutportName__18__/1
  m_2/1 -> __UniqueOutportName__19__/1
  t_1/1 -> __UniqueOutportName__20__/1
  t_2/1 -> __UniqueOutportName__21__/1
  t_dot_1/1 -> __UniqueOutportName__22__/1
  t_dot_2/1 -> __UniqueOutportName__23__/1
  E_1/1 -> __UniqueOutportName__24__/1
  E_2/1 -> __UniqueOutportName__25__/1
  Gs_1/1 -> __UniqueOutportName__26__/1
  Gs_2/1 -> __UniqueOutportName__27__/1

== system complete_model/ROBOT/Subsystem/MATLAB Function1/__OutputSSForSFun__ ==
  __UniqueInportName__1__ : Inport
  __UniqueInportName__2__ : Inport  Port=2
  __UniqueInportName__3__ : Inport  Port=3
  B_matrix : Outport
  G_matrix : Outport  Port=2
  C_matrix : Outport  Port=3
  wires:
  __UniqueInportName__1__/1 -> B_matrix/1  "B_matrix"
  __UniqueInportName__2__/1 -> G_matrix/1  "G_matrix"
  __UniqueInportName__3__/1 -> C_matrix/1  "C_matrix"

== matlab function complete_model/CONTROLLER/Subsystem1/Subsystem/MATLAB Function ==
  data: e_dot input; e input; q_ddot_ref input; q_dot input; C input; y output; B input; G input; D input; Kv input; Kd input
function y = fcn(e_dot,e,q_ddot_ref,q_dot,C, B , G , D, Kv , Kd)
    y =  + B * ( q_ddot_ref - Kv * e_dot + Kd * e) - ( C + D ) * q_dot - G  ;

== matlab function complete_model/CONTROLLER/Subsystem2/MATLAB Function ==
  data: E_1 input; E_2 input; Gs_1 input; Gs_2 input; Ix_1 input; Ix_2 input; Iy_1 input; Iy_2 input; Iz_1 input; Iz_2 input; b_1 input; b_2 input; g input; k_1 input; k_2 input; l_1 input; l_2 input; m_1 input; m_2 input; t_1 input; t_2 input; G_g output
function G_g  = fcn(E_1,E_2,Gs_1,Gs_2,Ix_1,Ix_2,Iy_1,Iy_2,Iz_1,Iz_2,b_1,b_2,g,k_1,k_2,l_1,l_2,m_1,m_2,t_1,t_2)
    G_g = G_grav(b_1,b_2,g,k_1,k_2,l_1,l_2,m_1,m_2,t_1);
